simulink model "PSO_LAB_CEP_ANFIS"  (R2020a)
settings: Solver=VariableStepAuto  StartTime=0.0  StopTime=20  RelTol=1e-3
libraries: fuzblock x1, powerlib x1
settings Model: Creator=Hp  LastModifiedBy=Hp

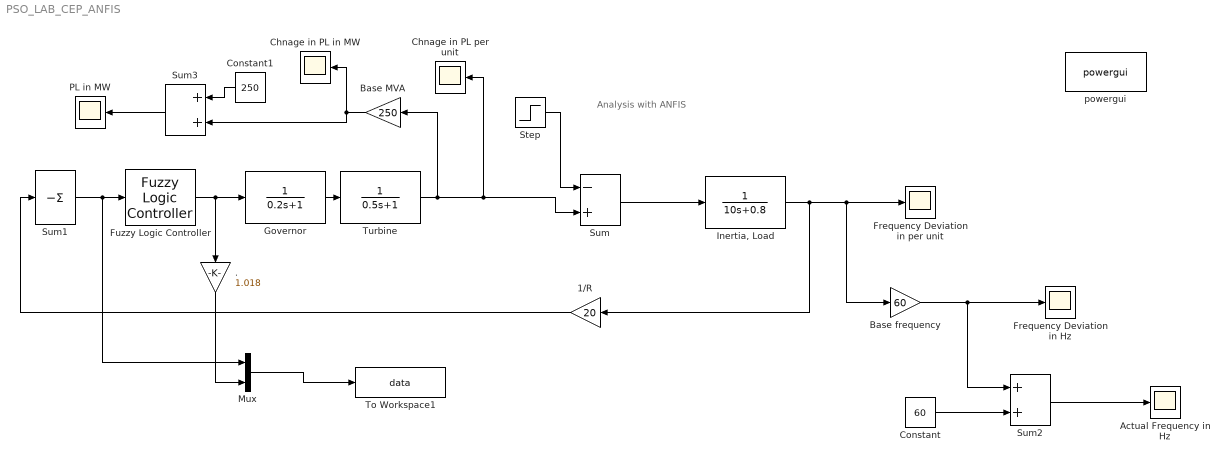
== system PSO_LAB_CEP_ANFIS ==
  note: Analysis with ANFIS
  . : Gain  Gain=1.018
  1/R : Gain  Gain=20
  Actual Frequency in Hz : Scope
  Base MVA : Gain  Gain=250
  Base frequency : Gain  Gain=60
  Chnage in PL in MW : Scope
  Chnage in PL per unit : Scope
  Constant : Constant  Value=60
  Constant1 : Constant  Value=250
  Frequency Deviation in Hz : Scope
  Frequency Deviation in per unit : Scope
  Fuzzy Logic Controller : fuzblock/Fuzzy Logic  Controller  FIS=LFCanfis  OutputSampleNumber=101  DataType=double  FuzzifiedInputs=off  RuleFiringStrengths=off  RuleOutputs=off  AggregatedOutputs=off  SimulateUsing=Interpreted execution  OutOfRangeInputValueMessage=warning  NoRuleFiredMessage=warning  EmptyOutputFuzzySetMessage=warning
  Governor : TransferFcn  Denominator=[0.2 1]
  "Inertia, Load" : TransferFcn  Denominator=[10 0.8]
  Mux : Mux  Inputs=2
  PL in MW : Scope
  Step : Step  Time=100  Before=0.2  After=0.2  SampleTime=0
  Sum : Sum  Inputs=-+
  Sum1 : Sum  Inputs=-
  Sum2 : Sum
  Sum3 : Sum
  To Workspace1 : ToWorkspace  VariableName=data  SampleTime=-1
  Turbine : TransferFcn  Denominator=[0.5 1]
  powergui : powerlib/powergui  Priority=1  SimulationMode=Continuous  SampleTime=50e-6  frequency=60  Iterations=50  frequencyindice=60  Pbase=100e6  ErrMax=1e-4  UnitsV=kV  UnitsW=MW  buscounter=0  FunctionMessages=off  echomessages=off  EnableUseOfTLC=off  CurrentSourceSwitches=off  DisableSnubberDevices=off  DisableRonSwitches=off  DisableVfSwitches=off  DisplayEquations=off  AutomaticDiscreteSolvers=off  SolverType=Tustin/Backward Euler (TBE)  Interpol=off  ExternalGateDelay=off  methode=off  Ts=100  x0status=blocks  SPID=on  SwTol=0  HookPort=off  NonlinearTolerance=1e-4  nMaxIteration=100  ContinueOnMaxIteration=off  RestoreLinks=warning  ResistiveCurrentMeasurement=off  Frange=[0:2:500]  Ylog=off  Xlog=on  ShowGrid=off  save=off  variable=ZData  structure=0  ZoomFFT=off  StartTime=0.0  cycles=1  DisplayStyle=1  fundamental=60  FreqAxis=off  MaxFrequency=1000  frequencyindicesteady=1  RmsSteady=1  display=off
  wires:
  Governor/1 -> Turbine/1
  Turbine/1 -> Base MVA/1, Chnage in PL per unit/1, Sum/2
  Step/1 -> Sum/1
  Sum/1 -> "Inertia, Load"/1
  "Inertia, Load"/1 -> Base frequency/1, Frequency Deviation in per unit/1, 1/R/1
  1/R/1 -> Sum1/1
  Base frequency/1 -> Sum2/1, Frequency Deviation in Hz/1
  Constant/1 -> Sum2/2
  Sum2/1 -> Actual Frequency in Hz/1
  Base MVA/1 -> Sum3/2, Chnage in PL in MW/1
  Constant1/1 -> Sum3/1
  Sum3/1 -> PL in MW/1
  Sum1/1 -> Fuzzy Logic Controller/1, Mux/1
  Fuzzy Logic Controller/1 -> Governor/1, ./1
  Mux/1 -> To Workspace1/1
  ./1 -> Mux/2
